simulink model "mpcVehicleSteering"  (R2017b)
settings: Solver=VariableStepAuto  StartTime=0.0  StopTime=10  RelTol=1e-3
undefined symbols (not defined in the file or in its folder): Ts, Vx
libraries: cstblocks x1, mpclib x1
settings Model: Creator=The MathWorks, Inc.  LastModifiedBy=rishi
settings CodeAppCC: StateflowObjectComments=on
settings SimscapeCC: SimscapeNormalizeSystem=off

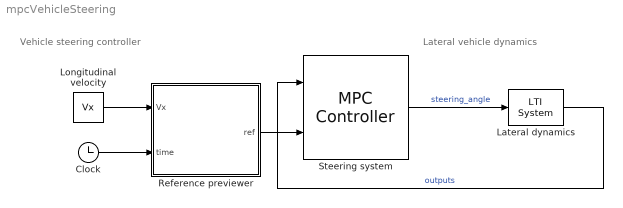
== system mpcVehicleSteering ==
  note: Lateral vehicle dynamics
  note: Vehicle steering controller
  Clock : Clock
  Lateral dynamics : cstblocks/LTI System  sys=vehicle  IC=[]
  Longitudinal velocity : Constant  Value=Vx  SampleTime=Ts
  Reference previewer : MATLAB Function  TreatAsAtomicUnit=on  SystemSampleTime=Ts
  Steering system : mpclib/MPC Controller  SCDEnableBlockLinearizationSpecification=on  mpcobj=mpc1  is_multiple=0  enable_value=0  return_u0=off  ref_from_ws=off  ref_signal_name=[]  ref_preview=off  md_from_ws=off  md_signal_name=[]  md_preview=off  from_project=off  project_file=MPCtask.mat  md_inport=off  mv_inport=off  cost_outport=off  return_sequence=off  return_qpstatus=off  return_state=off  state_inport=off  lims_inport=off  cc_inport=off  ywt_inport=off  is_designfromscratch=0  uwt_inport=off  duwt_inport=off  rhoeps_inport=off  uref_inport=off  n_ts=0.1  n_p=10  n_mv=1  n_md=0  n_ud=0  n_mo=2  n_uo=0  BlockDataType=double  SampleTimeInherited=off  switch_inport=off
  wires:
  Longitudinal velocity/1 -> Reference previewer/1(Vx)
  Steering system/1 -> Lateral dynamics/1  "steering_angle"
  Clock/1 -> Reference previewer/2(time)
  Reference previewer/1(ref) -> Steering system/2
  Lateral dynamics/1 -> Steering system/1  "outputs"

== matlab function mpcVehicleSteering/Reference previewer ==
  data: Vx input; time input; ref output
function ref = previewer(Vx,time)
% Get previewed reference trajectory

% Previw horizon is 10 sampling times (i.e. 10*0.1 = 1 seconds).
% Reference contains 2 signals (i.e. Y position and yaw angle).
ref = zeros(10,2); 

%% Previewing sequence
for ct = 1:10
   ref(ct,:) = doubleLaneChange(Vx,time + (ct-1)*0.1);
end
